simulink model "EBD"  (R2022b)
settings: Solver=VariableStepAuto  StartTime=0.0  StopTime=10  RelTol=1e-3
PreLoadFcn:
  | g = 9.81;
  | v0 = 27.77;
  | r_Roue = 0.3;
  | J = 0.5;
  | m = 1000;
  | 
  | Omega_0 = 0;
InitFcn:
  | ABS_config
values from neighbouring files (symbols this model uses):
  d = 1.5    [ABS_config.m]
  D = 3    [ABS_config.m]
  h = 0.7    [ABS_config.m]
libraries: simulink x2, slpidlib x2
settings Model: Creator=Youssef ABLALI  LastModifiedBy=Youssef ABLALI

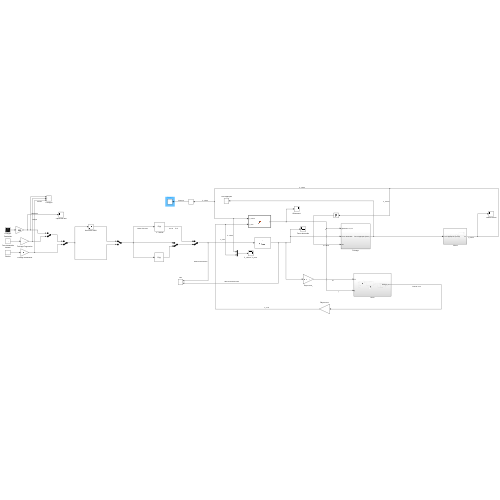
[thumbnail: Simulink's stored preview of the top-level diagram]
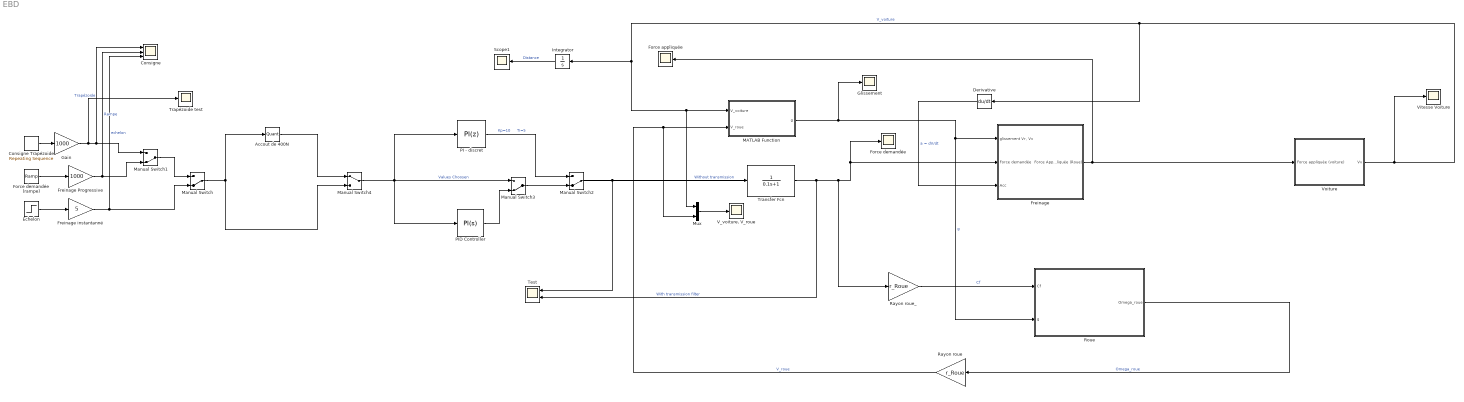
== system EBD ==
  "Accout de 400N " : Quantizer  QuantizationInterval=400
  Consigne : Scope  NumInputPorts=3
  Consigne Trapézoide : simulink/Sources/Repeating Sequence  rep_seq_t=[0 0.1 0.2 0.3 0.4 0.5]  rep_seq_y=[0 0 50 50 0 0]
  Derivative : Derivative
  Echelon : Step  After=2500  SampleTime=0
  Force appliquée : Scope
  Force demandée : Scope
  Force demandée (rampe) : simulink/Sources/Ramp  slope=1  start=0  InitialOutput=0
  Freinage : Subsystem
  Freinage Progressive : Gain  Gain=1000
  Freinage instantanné : Gain  Gain=5
  Gain : Gain  Gain=1000
  Glissement : Scope
  Integrator : Integrator
  MATLAB Function : MATLAB Function  TreatAsAtomicUnit=on
  Manual Switch{,1..3} (4 alike) : ManualSwitch  CurrentSetting=0
  Manual Switch4 : ManualSwitch
  Mux : Mux  Inputs=2
  PI - discret : slpidlib/PID Controller  Controller=PI  Form=Parallel  TimeDomain=Discrete-time  UseExternalTs=off  SampleTime=-1  IntegratorMethod=Forward Euler  FilterMethod=Forward Euler  ControllerParametersSource=internal  P=10  I=5  UseKiTs=off  D=0  N=100  UseFilter=on  TunerSelectOption=Transfer Function Based (PID Tuner App)  InitialConditionSource=internal  InitialConditionForIntegrator=0  InitialConditionForFilter=0  DifferentiatorICPrevScaledInput=0  ExternalReset=none  TrackingMode=off  Kt=1  LimitOutput=off  SatLimitsSource=internal  UpperSaturationLimit=inf  LowerSaturationLimit=-inf  LinearizeAsGain=off  AntiWindupMode=none  Kb=1  LimitIntegrator=off  UpperIntegratorSaturationLimit=inf  LowerIntegratorSaturationLimit=-inf  POutMin=[]  POutMax=[]  IOutMin=[]  IOutMax=[]  DOutMin=[]  DOutMax=[]  NOutMin=[]  NOutMax=[]  SumOutMin=[]  SumOutMax=[]  SaturationOutMin=[]  SaturationOutMax=[]  PParamMin=[]  PParamMax=[]  IParamMin=[]  IParamMax=[]  DParamMin=[]  DParamMax=[]  NParamMin=[]  NParamMax=[]  KbParamMin=[]  KbParamMax=[]  KtParamMin=[]  KtParamMax=[]  KbOutMin=[]  KbOutMax=[]  KtOutMin=[]  KtOutMax=[]  IntegratorOutMin=[]  IntegratorOutMax=[]  FilterOutMin=[]  FilterOutMax=[]  SumI1OutMin=[]  SumI1OutMax=[]  SumI2OutMin=[]  SumI2OutMax=[]  SumI3OutMin=[]  SumI3OutMax=[]  SumI4OutMin=[]  SumI4OutMax=[]  SumDOutMin=[]  SumDOutMax=[]  DifferentiatorOutMin=[]  DifferentiatorOutMax=[]  FilterDiffOutCoefMin=[]  FilterDiffOutCoefMax=[]  ReciprocalOutMin=[]  ReciprocalOutMax=[]  SumDenOutMin=[]  SumDenOutMax=[]  SumNumOutMin=[]  SumNumOutMax=[]  DivideOutMin=[]  DivideOutMax=[]  UdiffTsProdOutMin=[]  UdiffTsProdOutMax=[]  NTsProdOutMin=[]  NTsProdOutMax=[]  UintegralTsProdOutMin=[]  UintegralTsProdOutMax=[]  UngainTsProdOutMin=[]  UngainTsProdOutMax=[]  ClampingZeroOutDataTypeStr=Inherit: Inherit via back propagation  ClampingZeroOutMin=[]  ClampingZeroOutMax=[]  FilterDenConstantOutDataTypeStr=Inherit: Inherit via back propagation  FilterDenConstantOutMin=[]  FilterDenConstantOutMax=[]  PCopyOutDataTypeStr=Inherit: Inherit via back propagation  PCopyOutMin=[]  PCopyOutMax=[]  NCopyOutDataTypeStr=Inherit: Inherit via back propagation  NCopyOutMin=[]  NCopyOutMax=[]  IntegratorContinuousStateAttributes=''  IntegratorStateMustResolveToSignalObject=off  IntegratorRTWStateStorageClass=Auto  FilterContinuousStateAttributes=''  FilterStateMustResolveToSignalObject=off  FilterRTWStateStorageClass=Auto  ParallelPVariant=InternalParameters  IdealPVariant=Disabled  IVariant=InternalParameters  DVariant=Disabled  IntegratorVariant=Discrete  SatVariant=Disabled  AWVariant=Passthrough  PCopyVariant=Disabled  TRVariant=Disabled  FdbkBlocksVariant=Forward  IdealPFdbkVariant=Disabled  SatFdbkVariant=Disabled  DerivativeFilterVariant=Disabled  NVariant=Disabled  NCopyVariant=Disabled_SignalSpec  FilterICVariant=Disabled  IntegratorICVariant=InternalICs  ExternalResetVariant=Disabled  TRSumVariant=Passthrough  SumFdbkVariant=Disabled  SumVariant=Sum_PI  TsampFilterVariant=InternalTs  TsampNgainVariant=Passthrough  TsampIntegralVariant=Passthrough  ExternalSaturationOutDataTypeStr=Inherit: Same as second input
      settings: LibrarySourceBlock=simulink/Discrete/Discrete PID Controller
  PID Controller : slpidlib/PID Controller  Controller=PI  Form=Parallel  TimeDomain=Continuous-time  UseExternalTs=off  SampleTime=-1  IntegratorMethod=Forward Euler  FilterMethod=Forward Euler  ControllerParametersSource=internal  P=10  I=0.1  UseKiTs=off  D=3  N=100  UseFilter=on  TunerSelectOption=Transfer Function Based (PID Tuner App)  InitialConditionSource=internal  InitialConditionForIntegrator=0  InitialConditionForFilter=0  DifferentiatorICPrevScaledInput=0  ExternalReset=none  TrackingMode=off  Kt=1  LimitOutput=off  SatLimitsSource=internal  UpperSaturationLimit=inf  LowerSaturationLimit=-inf  LinearizeAsGain=on  AntiWindupMode=none  Kb=1  LimitIntegrator=off  UpperIntegratorSaturationLimit=inf  LowerIntegratorSaturationLimit=-inf  POutMin=[]  POutMax=[]  IOutMin=[]  IOutMax=[]  DOutMin=[]  DOutMax=[]  NOutMin=[]  NOutMax=[]  SumOutMin=[]  SumOutMax=[]  SaturationOutMin=[]  SaturationOutMax=[]  PParamMin=[]  PParamMax=[]  IParamMin=[]  IParamMax=[]  DParamMin=[]  DParamMax=[]  NParamMin=[]  NParamMax=[]  KbParamMin=[]  KbParamMax=[]  KtParamMin=[]  KtParamMax=[]  KbOutMin=[]  KbOutMax=[]  KtOutMin=[]  KtOutMax=[]  IntegratorOutMin=[]  IntegratorOutMax=[]  FilterOutMin=[]  FilterOutMax=[]  SumI1OutMin=[]  SumI1OutMax=[]  SumI2OutMin=[]  SumI2OutMax=[]  SumI3OutMin=[]  SumI3OutMax=[]  SumI4OutMin=[]  SumI4OutMax=[]  SumDOutMin=[]  SumDOutMax=[]  DifferentiatorOutMin=[]  DifferentiatorOutMax=[]  FilterDiffOutCoefMin=[]  FilterDiffOutCoefMax=[]  ReciprocalOutMin=[]  ReciprocalOutMax=[]  SumDenOutMin=[]  SumDenOutMax=[]  SumNumOutMin=[]  SumNumOutMax=[]  DivideOutMin=[]  DivideOutMax=[]  UdiffTsProdOutMin=[]  UdiffTsProdOutMax=[]  NTsProdOutMin=[]  NTsProdOutMax=[]  UintegralTsProdOutMin=[]  UintegralTsProdOutMax=[]  UngainTsProdOutMin=[]  UngainTsProdOutMax=[]  ClampingZeroOutDataTypeStr=Inherit: Inherit via back propagation  ClampingZeroOutMin=[]  ClampingZeroOutMax=[]  FilterDenConstantOutDataTypeStr=Inherit: Inherit via back propagation  FilterDenConstantOutMin=[]  FilterDenConstantOutMax=[]  PCopyOutDataTypeStr=Inherit: Inherit via back propagation  PCopyOutMin=[]  PCopyOutMax=[]  NCopyOutDataTypeStr=Inherit: Inherit via back propagation  NCopyOutMin=[]  NCopyOutMax=[]  IntegratorContinuousStateAttributes=''  IntegratorStateMustResolveToSignalObject=off  IntegratorRTWStateStorageClass=Auto  FilterContinuousStateAttributes=''  FilterStateMustResolveToSignalObject=off  FilterRTWStateStorageClass=Auto  ParallelPVariant=InternalParameters  IdealPVariant=Disabled  IVariant=InternalParameters  DVariant=Disabled  IntegratorVariant=Continuous  SatVariant=Disabled  AWVariant=Passthrough  PCopyVariant=Disabled  TRVariant=Disabled  FdbkBlocksVariant=Forward  IdealPFdbkVariant=Disabled  SatFdbkVariant=Disabled  DerivativeFilterVariant=Disabled  NVariant=Disabled  NCopyVariant=Disabled_SignalSpec  FilterICVariant=Disabled  IntegratorICVariant=InternalICs  ExternalResetVariant=Disabled  TRSumVariant=Passthrough  SumFdbkVariant=Disabled  SumVariant=Sum_PI  TsampFilterVariant=InternalTs  TsampNgainVariant=Passthrough  TsampIntegralVariant=Passthrough  ExternalSaturationOutDataTypeStr=Inherit: Same as second input
  Rayon roue : Gain  Gain=r_Roue
  Rayon roue_ : Gain  Gain=r_Roue
  Roue : Subsystem
  Scope1 : Scope
  Test : Scope  NumInputPorts=2
  Transfer Fcn : TransferFcn  Denominator=[0.1 1]
  Trapézoide test : Scope
  "V_voiture, V_roue" : Scope
  Vitesse Voiture : Scope
  Voiture : Subsystem
  wires:
  Freinage/1(Force Appliquée (Roue)) -> Voiture/1(Force appliquée (voiture)), Force appliquée/1
  Voiture/1("Vv ") -> Derivative/1, Integrator/1, Mux/1, MATLAB Function/1(V_voiture), Vitesse Voiture/1  "V_voiture"
  Rayon roue_/1 -> Roue/1(Cf)  "Cf"
  MATLAB Function/1(g) -> Glissement/1, Roue/2(g), Freinage/1("glissement Vr, Vv")  "g"
  Roue/1(Omega_roue) -> Rayon roue/1  "Omega_roue"
  Manual Switch1/1 -> Manual Switch/1
  Echelon/1 -> Freinage instantanné/1
  Force demandée (rampe)/1 -> Freinage Progressive/1
  Consigne Trapézoide/1 -> Gain/1
  Rayon roue/1 -> Mux/2, MATLAB Function/2(V_roue)  "V_roue"
  Gain/1 -> Trapézoide test/1, Consigne/1, Manual Switch1/1  "Trapézoide"
  Freinage Progressive/1 -> Consigne/2, Manual Switch1/2  "Rampe"
  Freinage instantanné/1 -> Manual Switch/2, Consigne/3  "echelon"
  Mux/1 -> "V_voiture, V_roue"/1
  Transfer Fcn/1 -> Test/2, Freinage/2(Force demandée), Force demandée/1, Rayon roue_/1  "With transmission filter"
  Manual Switch4/1 -> PID Controller/1, PI - discret/1, Manual Switch3/1  "Values Choosen"
  Manual Switch2/1 -> Test/1, Transfer Fcn/1  "Without transmission"
  Manual Switch3/1 -> Manual Switch2/2
  PID Controller/1 -> Manual Switch3/2
  PI - discret/1 -> Manual Switch2/1  "Kp=10     Ti=5"
  Integrator/1 -> Scope1/1  "Distance"
  Manual Switch/1 -> "Accout de 400N "/1, Manual Switch4/2
  "Accout de 400N "/1 -> Manual Switch4/1
  Derivative/1 -> Freinage/3(Acc)  "a = dV/dt"

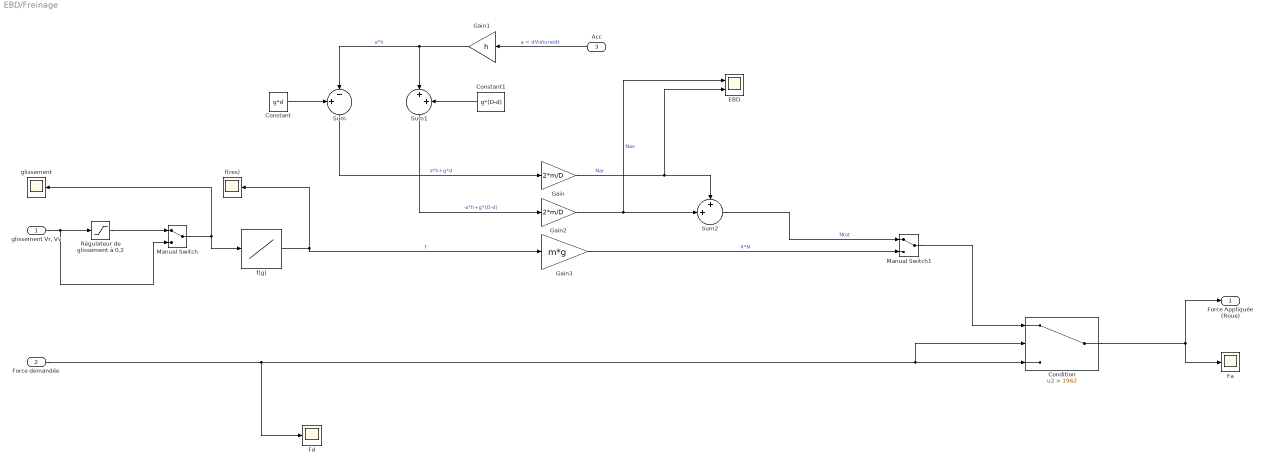
== system EBD/Freinage ==
  "glissement Vr, Vv" : Inport
  Force demandée : Inport  Port=2
  Acc : Inport  Port=3
  "Condition " : Switch  Criteria=u2 > Threshold  Threshold=1962  SaturateOnIntegerOverflow=off  InputSameDT=off
  Constant : Constant  Value=g*d
  Constant1 : Constant  Value=g*(D-d)
  EBD : Scope  NumInputPorts=2
  "Fa " : Scope
  Fd : Scope
  Gain : Gain  Gain=2*m/D
  Gain1 : Gain  Gain=h
  Gain2 : Gain  Gain=2*m/D
  Gain3 : Gain  Gain=m*g
  Manual Switch : ManualSwitch
  Manual Switch1 : ManualSwitch
  Régulateur de glissement à 0.2 : Saturate  UpperLimit=0.2  LowerLimit=0
  Sum : Sum  Inputs=+-|
  Sum1 : Sum  Inputs=|++
  Sum2 : Sum  Inputs=++|
  f(g) : Lookup_n-D  NumberOfTableDimensions=1  BreakpointsForDimension1=[0,0.1,0.2,0.3,0.4,0.5,0.6,0.7,0.8,0.9,1.0]  Table=[0.0,0.85,0.95,0.78,0.73,0.7,0.68,0.66,0.64,0.62,0.61]  InternalRulePriority=Speed  RndMeth=Simplest
  f(res) : Scope
  glissement : Scope
  Force Appliquée (Roue) : Outport  VectorParamsAs1DForOutWhenUnconnected=off
  wires:
  "Condition "/1 -> Force Appliquée (Roue)/1, "Fa "/1
  f(g)/1 -> Gain3/1, f(res)/1  "f"
  Force demandée/1 -> "Condition "/3, "Condition "/2, Fd/1
  Manual Switch/1 -> f(g)/1, glissement/1
  Régulateur de glissement à 0.2/1 -> Manual Switch/1
  "glissement Vr, Vv"/1 -> Manual Switch/2, Régulateur de glissement à 0.2/1
  Acc/1 -> Gain1/1  "a = dVoiture/dt"
  Constant/1 -> Sum/1
  Gain1/1 -> Sum/2, Sum1/1  "a*h"
  Sum/1 -> Gain/1  "a*h+g*d"
  Gain/1 -> EBD/2, Sum2/1  "Nar"
  Constant1/1 -> Sum1/2
  Sum1/1 -> Gain2/1  "-a*h+g*(D-d)"
  Gain2/1 -> EBD/1, Sum2/2  "Nav"
  Sum2/1 -> Manual Switch1/1  "Ntot"
  Gain3/1 -> Manual Switch1/2  "4*N"
  Manual Switch1/1 -> "Condition "/1

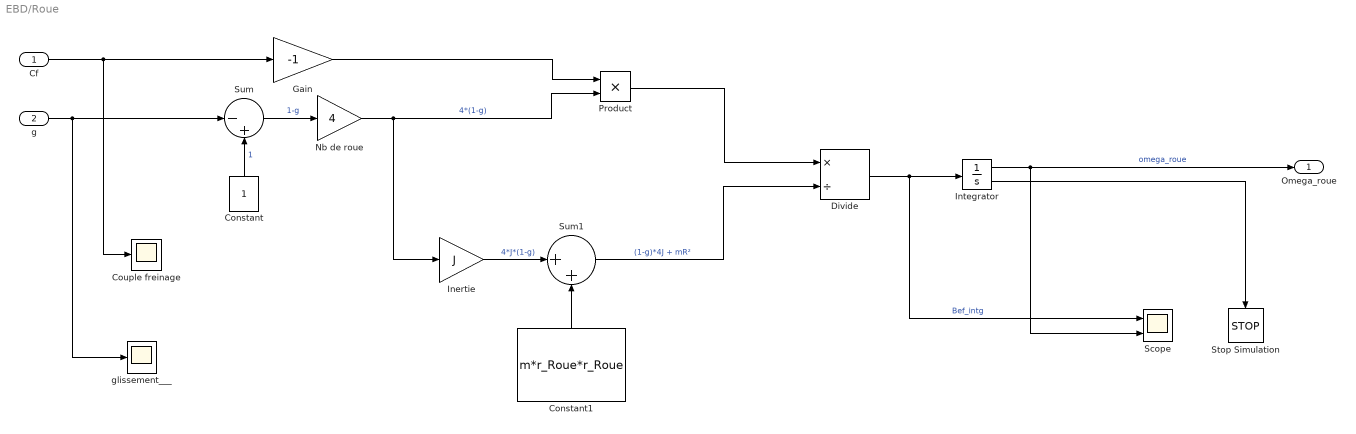
== system EBD/Roue ==
  Cf : Inport
  g : Inport  Port=2
  Constant : Constant
  Constant1 : Constant  Value=m*r_Roue*r_Roue
  Couple freinage : Scope
  Divide : Product  Inputs=*/
  Gain : Gain  Gain=-1
  Inertie : Gain  Gain=J
  Integrator : Integrator  InitialCondition=Omega_0  LimitOutput=on  LowerSaturationLimit=0  ShowSaturationPort=on
  Nb de roue : Gain  Gain=4
  Product : Product
  Scope : Scope  NumInputPorts=2
  Stop Simulation : Stop
  Sum : Sum  Inputs=|-+
  Sum1 : Sum  Inputs=|++
  glissement___ : Scope
  Omega_roue : Outport
  wires:
  Inertie/1 -> Sum1/1  "4*J*(1-g)"
  Sum/1 -> Nb de roue/1  "1-g"
  Sum1/1 -> Divide/2  "(1-g)*4J + mR²"
  Constant1/1 -> Sum1/2
  Product/1 -> Divide/1
  Constant/1 -> Sum/2  "1"
  Divide/1 -> Scope/1, Integrator/1  "Bef_intg"
  Nb de roue/1 -> Inertie/1, Product/2  "4*(1-g)"
  g/1 -> glissement___/1, Sum/1
  Cf/1 -> Couple freinage/1, Gain/1
  Integrator/1 -> Scope/2, Omega_roue/1  "omega_roue"
  Gain/1 -> Product/1
  Integrator/2 -> Stop Simulation/1

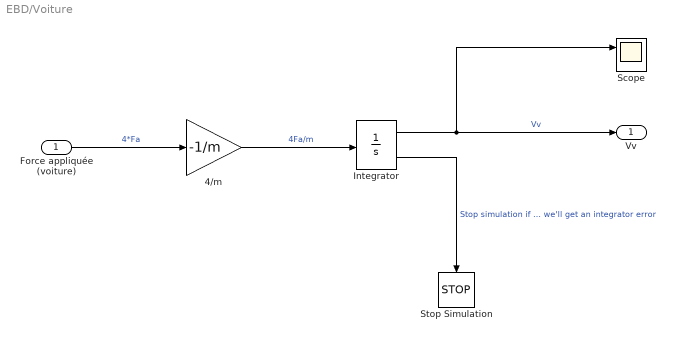
== system EBD/Voiture ==
  Force appliquée (voiture) : Inport
  4/m : Gain  Gain=-1/m
  Integrator : Integrator  InitialCondition=v0  LimitOutput=on  LowerSaturationLimit=0  ShowSaturationPort=on
  Scope : Scope  NumInputPorts=2
  Stop Simulation : Stop
  "Vv " : Outport
  wires:
  Force appliquée (voiture)/1 -> 4/m/1  "4*Fa"
  4/m/1 -> Integrator/1  "4Fa/m"
  Integrator/1 -> Scope/1, "Vv "/1  "Vv"
  Integrator/2 -> Stop Simulation/1  "Stop simulation if 0 is reached otherwise, we'll get an integrator error"

== matlab function EBD/MATLAB Function ==
  data: V_voiture input; V_roue input; g output
function g = fcn(V_voiture,V_roue)

g = (V_voiture - V_roue)/V_voiture;
